simulink model "ProblemState_RL"  (R2025b)
settings: Solver=ode4  StartTime=0.0  StopTime=1000  FixedStep=Ts  RelTol=1e-3
undefined symbols (not defined in the file): DiscIntNeverNeededParam, sigbuilder_block, Ts
libraries: slpidlib x1, rllib x1
settings Model: Creator=goelp4  LastModifiedBy=msi
settings OptimizationCC: BlockReduction=off  DefaultParameterBehavior=Inlined  BufferReuse=off
settings DebuggingCC: UnconnectedInputMsg=warning  UnconnectedOutputMsg=warning  UnconnectedLineMsg=warning
settings ModelReferenceCC: EnableRefExpFcnMdlSchedulingChecks=on
settings RTWCC: GPUComputeCapability=3.5  DLArmComputeVersion=19.05

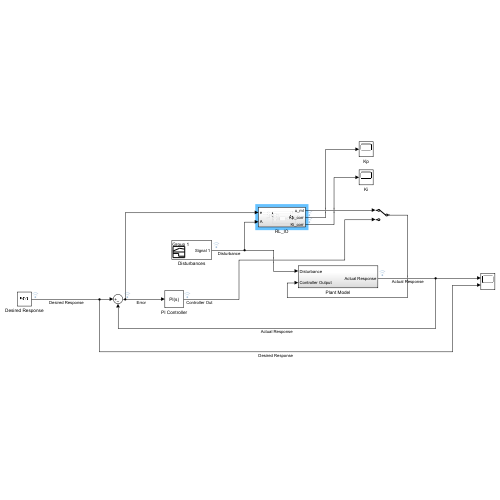
[thumbnail: Simulink's stored preview of the top-level diagram]
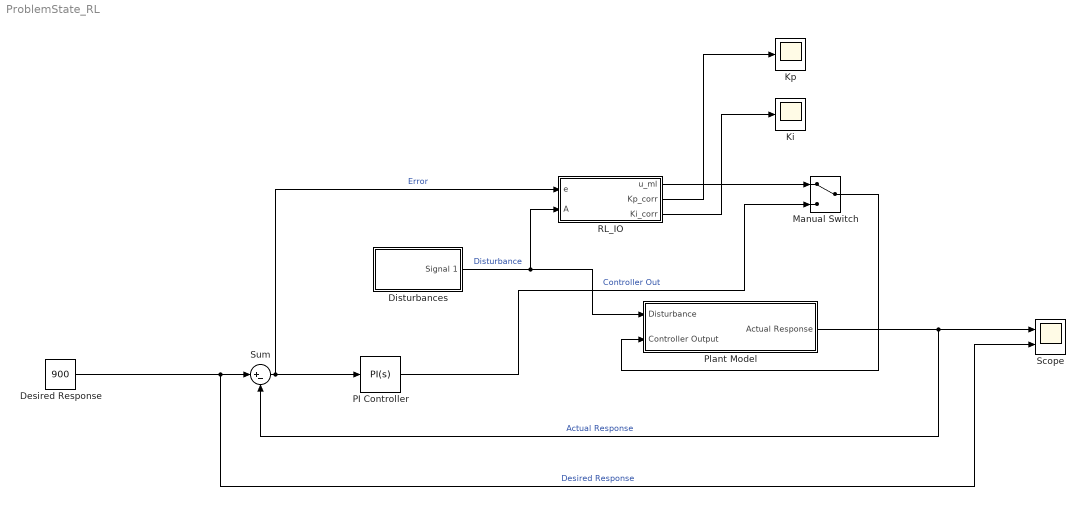
== system ProblemState_RL ==
  Desired Response : Constant  Value=900
  Disturbances : Subsystem  Tag=STV Subsys  LoadFcn=sigbuilder_block('load');  StartFcn=sigbuilder_block('start');  StopFcn=sigbuilder_block('stop');  ClipboardFcn=sigbuilder_block('clipboard');  mask(Sigbuilder block){tuvar=[0:10]}
      mask help: Simulink:masks:SigbuilderBlock_MD
      mask init:
      | if ~strcmp(get_param(bdroot(gcbh),'SimulationStatus'),'stopped') tuvar = sigbuilder_block('maskInit'); end
      settings: CopyFcn=sigbuilder_block('copy');  DeleteFcn=sigbuilder_block('delete');  ModelCloseFcn=sigbuilder_block('modelClose');  PreSaveFcn=sigbuilder_block('preSave');  PauseFcn=sigbuilder_block('pause');  ContinueFcn=sigbuilder_block('continue');  NameChangeFcn=sigbuilder_block('namechange');  OpenFcn=sigbuilder_block('open',[252.75 107.25 644.25 387.75 ]);  CloseFcn=sigbuilder_block('close');
      mask Display: plot(0, 0, 100, 100,[2, 2, 32, 32, 2], [68, 8, 8, 68, 68],[32, 2], [38, 38], [32, 19, 2],[53, 60, 44], [32, 17, 17, 2],[16, 16, 31, 31]);txt = getActiveGroup(gcbh);text(2, 100, txt,'verticalAlignment', 'top');
  Ki : Scope
  Kp : Scope
      settings: DataLoggingVariableName=ScopeData2
  Manual Switch : ManualSwitch
  PI Controller : slpidlib/PID Controller  Controller=PI  Form=Parallel  TimeDomain=Continuous-time  UseExternalTs=off  SampleTime=-1  IntegratorMethod=Forward Euler  FilterMethod=Forward Euler  ControllerParametersSource=internal  P=1  I=1  UseKiTs=off  D=0  UseExternalDerivativeSource=off  N=100  UseFilter=on  TunerSelectOption=Transfer Function Based (PID Tuner App)  InitialConditionSource=internal  InitialConditionForIntegrator=0  InitialConditionForFilter=0  DifferentiatorICPrevScaledInput=0  ExternalReset=none  TrackingMode=off  Kt=1  LimitOutput=off  SatLimitsSource=internal  UpperSaturationLimit=inf  LowerSaturationLimit=-inf  LinearizeAsGain=on  AntiWindupMode=none  Kb=1  LimitIntegrator=off  UpperIntegratorSaturationLimit=inf  LowerIntegratorSaturationLimit=-inf  POutMin=[]  POutMax=[]  IOutMin=[]  IOutMax=[]  DOutMin=[]  DOutMax=[]  NOutMin=[]  NOutMax=[]  SumOutMin=[]  SumOutMax=[]  SaturationOutMin=[]  SaturationOutMax=[]  PParamMin=[]  PParamMax=[]  IParamMin=[]  IParamMax=[]  DParamMin=[]  DParamMax=[]  NParamMin=[]  NParamMax=[]  KbParamMin=[]  KbParamMax=[]  KtParamMin=[]  KtParamMax=[]  KbOutMin=[]  KbOutMax=[]  KtOutMin=[]  KtOutMax=[]  IntegratorOutMin=[]  IntegratorOutMax=[]  FilterOutMin=[]  FilterOutMax=[]  SumI1OutMin=[]  SumI1OutMax=[]  SumI2OutMin=[]  SumI2OutMax=[]  SumI3OutMin=[]  SumI3OutMax=[]  SumI4OutMin=[]  SumI4OutMax=[]  SumDOutMin=[]  SumDOutMax=[]  DifferentiatorOutMin=[]  DifferentiatorOutMax=[]  FilterDiffOutCoefMin=[]  FilterDiffOutCoefMax=[]  ReciprocalOutMin=[]  ReciprocalOutMax=[]  SumDenOutMin=[]  SumDenOutMax=[]  SumNumOutMin=[]  SumNumOutMax=[]  DivideOutMin=[]  DivideOutMax=[]  UdiffTsProdOutMin=[]  UdiffTsProdOutMax=[]  NTsProdOutMin=[]  NTsProdOutMax=[]  UintegralTsProdOutMin=[]  UintegralTsProdOutMax=[]  UngainTsProdOutMin=[]  UngainTsProdOutMax=[]  ClampingZeroOutDataTypeStr=Inherit: Inherit via back propagation  ClampingZeroOutMin=[]  ClampingZeroOutMax=[]  FilterDenConstantOutDataTypeStr=Inherit: Inherit via back propagation  FilterDenConstantOutMin=[]  FilterDenConstantOutMax=[]  PCopyOutDataTypeStr=Inherit: Inherit via back propagation  PCopyOutMin=[]  PCopyOutMax=[]  NCopyOutDataTypeStr=Inherit: Inherit via back propagation  NCopyOutMin=[]  NCopyOutMax=[]  IntegratorContinuousStateAttributes=''  IntegratorStateMustResolveToSignalObject=off  IntegratorRTWStateStorageClass=Auto  FilterContinuousStateAttributes=''  FilterStateMustResolveToSignalObject=off  FilterRTWStateStorageClass=Auto  ParallelPVariant=InternalParameters  IdealPVariant=Disabled  IVariant=InternalParameters  DVariant=Disabled  IntegratorVariant=Continuous  SatVariant=Disabled  AWVariant=Passthrough  PCopyVariant=Disabled  TRVariant=Disabled  FdbkBlocksVariant=Forward  IdealPFdbkVariant=Disabled  SatFdbkVariant=Disabled  DerivativeFilterVariant=Disabled  NVariant=Disabled  NCopyVariant=Disabled_SignalSpec  FilterICVariant=Disabled  IntegratorICVariant=InternalICs  ExternalResetVariant=Disabled  TRSumVariant=Passthrough  SumFdbkVariant=Disabled  SumVariant=Sum_PI  TsampFilterVariant=InternalTs  TsampNgainVariant=Passthrough  TsampIntegralVariant=Disabled_SignalSpec  ExternalSaturationOutDataTypeStr=Inherit: Same as second input  DerivativeSourceVariant=Disabled  PreIntVariant=InternalPreInt
  Plant Model : Subsystem
  RL_IO : Subsystem
  Scope : Scope  NumInputPorts=2
  Sum : Sum  Inputs=|+-
  wires:
  Desired Response/1 -> Sum/1, Scope/2  "Desired Response"
  Plant Model/1(Actual Response) -> Sum/2, Scope/1  "Actual Response"
  Sum/1 -> RL_IO/1(e), PI Controller/1  "Error"
  Disturbances/1(Signal 1) -> RL_IO/2(A), Plant Model/1(Disturbance)  "Disturbance"
  RL_IO/1(u_ml) -> Manual Switch/1
  PI Controller/1 -> Manual Switch/2  "Controller Out"
  Manual Switch/1 -> Plant Model/2(Controller Output)
  RL_IO/2(Kp_corr) -> Kp/1
  RL_IO/3(Ki_corr) -> Ki/1

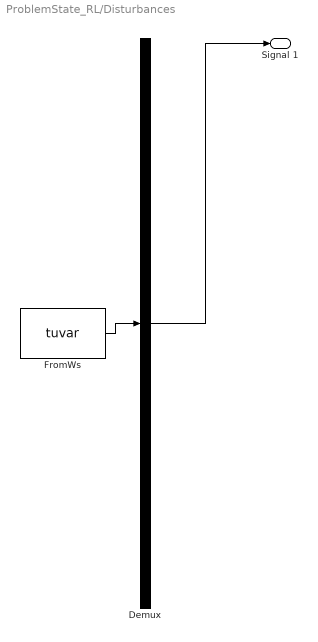
== system ProblemState_RL/Disturbances ==
  Demux : Demux  Tag=STV Demux  Outputs=1
      settings: DisplayOption=none
  FromWs : FromWorkspace  Tag=STV FromWs  VariableName=tuvar
      SigBuilderData=|
      | common.afterFinalStr = 'Extrapolate'
      | common.sampleTime = 0
      | dataSet.timeRange = [0 1000]
      | dataSet.name = 'Group 1'
      | sbobj.Groups.Name = 'Group 1'
      | sbobj.Groups.Signals.Name = 'Signal 1'
      | sbobj.Groups.Signals.XData = [0 2 3 4 5 6 7 8 9 10 11 12 ... (1000 elements, 1x1000)]
      | sbobj.Groups.Signals.YData = [0 0 0 0 0 0 0 0 0 0 0 0 ... (1000 elements, 1x1000)]
      | sbobj.Groups.TimeRange = [0 1000]
  Signal 1 : Outport  Tag=STV Outport
  wires:
  Demux/1 -> Signal 1/1
  FromWs/1 -> Demux/1

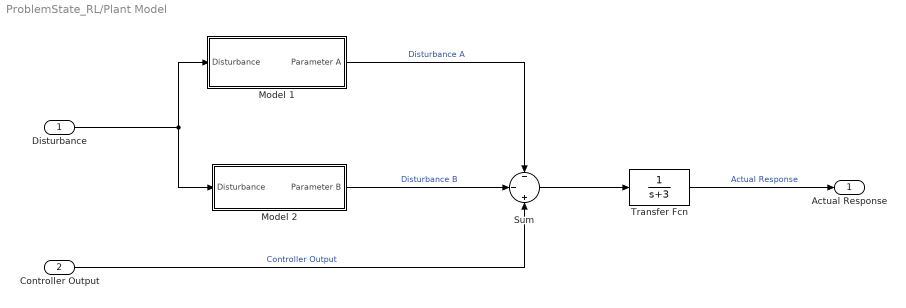
== system ProblemState_RL/Plant Model ==
  Disturbance : Inport
  Controller Output : Inport  Port=2
  Model 1 : Subsystem
  Model 2 : Subsystem
  Sum : Sum  Inputs=-|-|+
  Transfer Fcn : TransferFcn  Denominator=[1 3]
  Actual Response : Outport
  wires:
  Transfer Fcn/1 -> Actual Response/1  "Actual Response"
  Sum/1 -> Transfer Fcn/1
  Disturbance/1 -> Model 2/1(Disturbance), Model 1/1(Disturbance)
  Controller Output/1 -> Sum/3  "Controller Output"
  Model 2/1(Parameter B) -> Sum/2  "Disturbance B"
  Model 1/1(Parameter A) -> Sum/1  "Disturbance A"

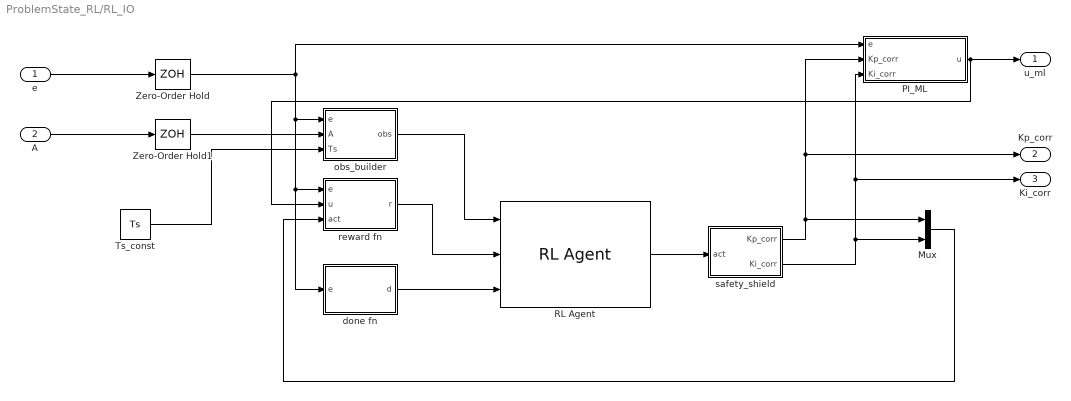
== system ProblemState_RL/RL_IO ==
  e : Inport
  A : Inport  Port=2
  Mux : Mux  Inputs=2
  PI_ML : Subsystem
  RL Agent : rllib/RL Agent  Agent=agentObj  ExternalActionAsInput=off  ProvideLastAction=off  ProvideCumRwd=off  TreatAsDirectFeedthrough=on  UseStrictObservationDataTypes=off
  Ts_const : Constant  Value=Ts
  Zero-Order Hold : ZeroOrderHold  SampleTime=Ts
  Zero-Order Hold1 : ZeroOrderHold  SampleTime=Ts
  done fn : MATLAB Function  TreatAsAtomicUnit=on
  obs_builder : MATLAB Function  TreatAsAtomicUnit=on
  reward fn : MATLAB Function  TreatAsAtomicUnit=on
  safety_shield : MATLAB Function  TreatAsAtomicUnit=on
  u_ml : Outport
  Kp_corr : Outport  Port=2
  Ki_corr : Outport  Port=3
  wires:
  e/1 -> Zero-Order Hold/1
  A/1 -> Zero-Order Hold1/1
  RL Agent/1 -> safety_shield/1(act)
  obs_builder/1(obs) -> RL Agent/1
  safety_shield/2(Ki_corr) -> Mux/2, PI_ML/3(Ki_corr), Ki_corr/1
  safety_shield/1(Kp_corr) -> Mux/1, PI_ML/2(Kp_corr), Kp_corr/1
  PI_ML/1(u) -> reward fn/2(u), u_ml/1
  reward fn/1(r) -> RL Agent/2
  done fn/1(d) -> RL Agent/3
  Mux/1 -> reward fn/3(act)
  Ts_const/1 -> obs_builder/3(Ts)
  Zero-Order Hold/1 -> done fn/1(e), reward fn/1(e), obs_builder/1(e), PI_ML/1(e)
  Zero-Order Hold1/1 -> obs_builder/2(A)

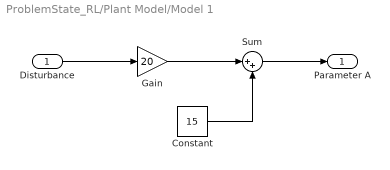
== system ProblemState_RL/Plant Model/Model 1 ==
  Disturbance : Inport
  Constant : Constant  Value=15
  Gain : Gain  Gain=20
  Sum : Sum  Inputs=|++
  Parameter A : Outport
  wires:
  Disturbance/1 -> Gain/1
  Gain/1 -> Sum/1
  Sum/1 -> Parameter A/1
  Constant/1 -> Sum/2

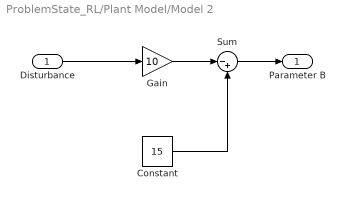
== system ProblemState_RL/Plant Model/Model 2 ==
  Disturbance : Inport
  Constant : Constant  Value=15
  Gain : Gain  Gain=10
  Sum : Sum  Inputs=|-+
  Parameter B : Outport
  wires:
  Disturbance/1 -> Gain/1
  Gain/1 -> Sum/1
  Sum/1 -> Parameter B/1
  Constant/1 -> Sum/2

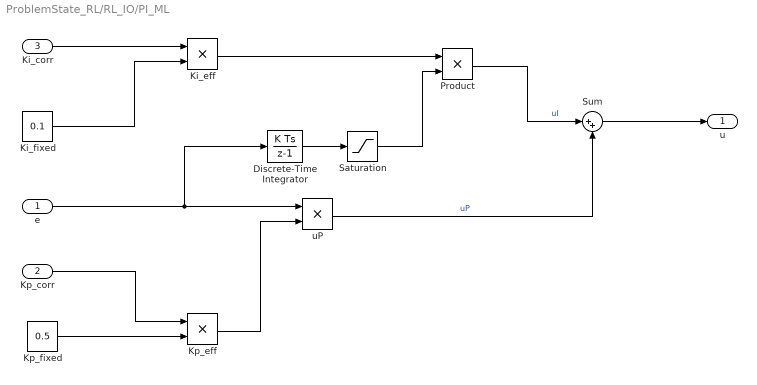
== system ProblemState_RL/RL_IO/PI_ML ==
  e : Inport
  Kp_corr : Inport  Port=2
  Ki_corr : Inport  Port=3
  Discrete-Time Integrator : DiscreteIntegrator  gainval=Ts  SampleTime=-1  ICPrevOutput=DiscIntNeverNeededParam  ICPrevScaledInput=DiscIntNeverNeededParam
  Ki_eff : Product
  Ki_fixed : Constant  Value=0.1
  Kp_eff : Product
  Kp_fixed : Constant  Value=0.5
  Product : Product
  Saturation : Saturate  UpperLimit=5e4  LowerLimit=-5e4
  Sum : Sum  Inputs=|++
  uP : Product
  u : Outport
  wires:
  Kp_fixed/1 -> Kp_eff/2
  Kp_corr/1 -> Kp_eff/1
  Ki_corr/1 -> Ki_eff/1
  Ki_fixed/1 -> Ki_eff/2
  e/1 -> uP/1, Discrete-Time Integrator/1
  Kp_eff/1 -> uP/2
  Discrete-Time Integrator/1 -> Saturation/1
  uP/1 -> Sum/2  "uP"
  Sum/1 -> u/1
  Ki_eff/1 -> Product/1
  Saturation/1 -> Product/2
  Product/1 -> Sum/1  "uI"

== matlab function ProblemState_RL/RL_IO/obs_builder ==
  settings: updateMethod=DISCRETE  sampleTime=Ts
  data: e input; obs output double size=[5 1]; A input; Ts input
function obs = obs_builder(e, A, Ts)
%#codegen
persistent e_prev A_prev ie

if isempty(e_prev)
    e_prev = 0;
    A_prev = 0;
    ie = 0;
end

de = (e - e_prev) / Ts;
dA = (A - A_prev) / Ts;

ie = ie + e * Ts;
ie = min(max(ie, -5e4), 5e4);

obs = zeros(5,1);
obs(1) = e;
obs(2) = A;
obs(3) = de;
obs(4) = ie;
obs(5) = dA;

e_prev = e;
A_prev = A;
end

== matlab function ProblemState_RL/RL_IO/reward fn ==
  settings: updateMethod=DISCRETE  sampleTime=Ts
  data: e input; u input; r output; act input
function r = reward_fn(e, u, act)

ref = 900;

persistent prevAbsE lastAct inBandCount
if isempty(prevAbsE)
    prevAbsE = abs(e);
    lastAct = [1; 1];
    inBandCount = 0;
end

act = act(:);

eAbs = abs(e);
eN   = eAbs / ref;
uN   = abs(u) / 1000;

progress = (prevAbsE - eAbs) / ref;

actMove = sum((act - lastAct).^2);
actMag  = sum((act - 1).^2);

r = ...
    + 3.0 * progress ...     % encourage reducing error quickly
    - 2.5 * eN ...           % strong error penalty
    - 0.01 * uN ...          % mild control effort penalty
    - 0.03 * actMove ...     % penalize sudden gain jumps
    - 0.002 * actMag;        % mild penalty on large gain corrections

% Overshoot penalty: if y > r, then e = r - y < 0
if e < 0
    r = r - 0.75 * abs(e) / ref;
end

% Band-based bonuses to encourage settling
if eAbs <= 0.01 * ref
    inBandCount = inBandCount + 1;
    r = r + 0.5;
else
    inBandCount = 0;
end

if eAbs <= 0.0025 * ref
    r = r + 1.0;
end

% Extra penalties for clearly bad behavior
if eAbs > 0.25 * ref
    r = r - 0.5;
end

if eAbs > 0.50 * ref
    r = r - 2.0;
end

% Bonus for staying in 1% band for a while
% With Ts = 0.05, 20 steps ~ 1 second
if inBandCount >= 20
    r = r + 1.0;
end

prevAbsE = eAbs;
lastAct = act;
end

== matlab function ProblemState_RL/RL_IO/done fn ==
  settings: updateMethod=DISCRETE  sampleTime=Ts
  data: e input; d output
function d = done_fn(e)
d = (abs(e) > 2*900);
end

== matlab function ProblemState_RL/RL_IO/safety_shield ==
  settings: updateMethod=DISCRETE  sampleTime=Ts
  data: act input; Kp_corr output; Ki_corr output
function [Kp_corr, Ki_corr] = safety_shield(act)

persistent last
if isempty(last)
    last = [1;1];
end

amin = [0.2; 0.2];
amax = [5.0; 5.0];
a = min(max(act(:), amin), amax);

dmax = [0.05; 0.05];
delta = a - last;
delta = min(max(delta, -dmax), dmax);
a = last + delta;

alpha = 0.8;
a = alpha*last + (1-alpha)*a;

Kp_corr = a(1);
Ki_corr = a(2);
last = a;
end
